simulink library "data_driven_lib_ctl"  (R2024a)
settings: Solver=VariableStepAuto  StartTime=0.0  StopTime=10.0  RelTol=1e-3
undefined symbols (not defined in the file or in its folder): ATDeePC_data, ATDeePC_DT, ATDeePC_LT, ATDeePC_PT, ATDeePC_trajectory_T, ATDeePC_tune_data, ATDeePC_tune_DT, ATDeePC_tune_input_T, ATDeePC_tune_LT, ATDeePC_tune_PT, ATDeePC_tune_trajectory_T, ATExplicitDeePC_data, ATExplicitDeePC_DT, ATExplicitDeePC_PT, DeePC_data, DeePC_DT, DeePC_LT, DeePC_PT, DeePCPI_data, DeePCPI_DT, DeePCPI_LT, DeePCPI_PT, ExplicitDeePC_data, ExplicitDeePC_DT, ExplicitDeePC_PT, ExplicitDeePCCodegen_data, ExplicitDeePCCodegen_DT, ExplicitDeePCCodegen_PT, extrinsic
libraries: otter_controllers x1
settings Model: Creator=luka  LastModifiedBy=luka

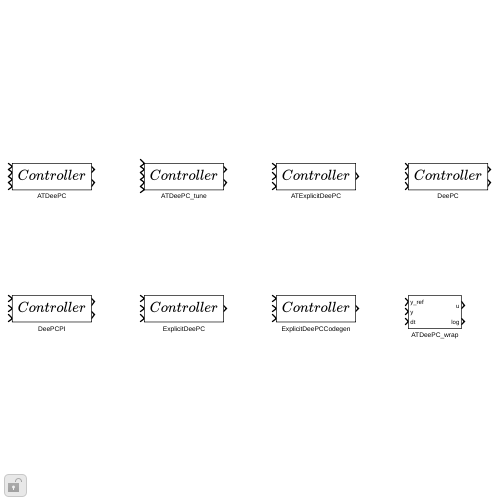
[thumbnail: Simulink's stored preview of the top-level diagram]
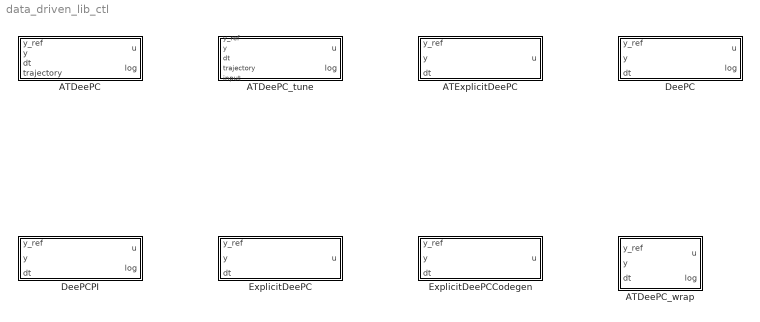
== system data_driven_lib_ctl ==
  ATDeePC : Subsystem  Tag=__cs_comptype:ctl;__cs_compimpl:mat;  mask{iid__=[0], pid__=[65 84 68 101 101 80 67 58 100 97 116 97 95 100 114 105 118 101 110 95 108 105 98], context_path=, params=[], LogEntryType=ATDeePC_LT, data=ATDeePC_data, ParamsType=ATDeePC_PT, DataType=ATDeePC_DT, u_ic=0, trajectory_T=ATDeePC_trajectory_T}
  ATDeePC_tune : Subsystem  Tag=__cs_comptype:ctl;__cs_compimpl:mat;  mask{iid__=[0], pid__=[65 84 68 101 101 80 67 95 116 117 110 101 58 100 97 116 97 95 100 114 105 118 101 110 95 108 105 98], context_path=, params=[], LogEntryType=ATDeePC_tune_LT, data=ATDeePC_tune_data, ParamsType=ATDeePC_tune_PT, DataType=ATDeePC_tune_DT, u_ic=0, trajectory_T=ATDeePC_tune_trajectory_T, input_T=ATDeePC_tune_input_T}
  ATDeePC_wrap : Subsystem  Tag=controller;__cs_comptype:ctl;__cs_compimpl:slx;  mask{trajectory_T=0, data=0, db_params=0, iid__=[0], pid__=[65 84 68 101 101 80 67 95 119 114 97 112 58 100 97 116 97 95 100 114 105 118 101 110 95 108 105 98], context_path=, params=[], params_struct_name=}
  ATExplicitDeePC : Subsystem  Tag=__cs_comptype:ctl;__cs_compimpl:mat;  mask{iid__=[0], pid__=[65 84 69 120 112 108 105 99 105 116 68 101 101 80 67 58 100 97 116 97 95 100 114 105 118 101 110 95 108 105 98], context_path=, params=[], data=ATExplicitDeePC_data, ParamsType=ATExplicitDeePC_PT, DataType=ATExplicitDeePC_DT, u_ic=0}
  DeePC : Subsystem  Tag=__cs_comptype:ctl;__cs_compimpl:mat;  mask{iid__=[0], pid__=[68 101 101 80 67 58 100 97 116 97 95 100 114 105 118 101 110 95 108 105 98], context_path=, params=[], LogEntryType=DeePC_LT, data=DeePC_data, ParamsType=DeePC_PT, DataType=DeePC_DT, u_ic=0}
  DeePCPI : Subsystem  Tag=__cs_comptype:ctl;__cs_compimpl:mat;  mask{iid__=[0], pid__=[68 101 101 80 67 80 73 58 100 97 116 97 95 100 114 105 118 101 110 95 108 105 98], context_path=, params=[], LogEntryType=DeePCPI_LT, data=DeePCPI_data, ParamsType=DeePCPI_PT, DataType=DeePCPI_DT, u_ic=0}
  ExplicitDeePC : Subsystem  Tag=__cs_comptype:ctl;__cs_compimpl:mat;  mask{iid__=[0], pid__=[69 120 112 108 105 99 105 116 68 101 101 80 67 58 100 97 116 97 95 100 114 105 118 101 110 95 108 105 98], context_path=, params=[], data=ExplicitDeePC_data, ParamsType=ExplicitDeePC_PT, DataType=ExplicitDeePC_DT, u_ic=0}
  ExplicitDeePCCodegen : Subsystem  Tag=__cs_comptype:ctl;__cs_compimpl:mat;  mask{iid__=[0], pid__=[69 120 112 108 105 99 105 116 68 101 101 80 67 67 111 100 101 103 101 110 58 100 97 116 97 95 100 114 105 118 101 110 95 108 105 98], context_path=, params=[], data=ExplicitDeePCCodegen_data, ParamsType=ExplicitDeePCCodegen_PT, DataType=ExplicitDeePCCodegen_DT, u_ic=0}

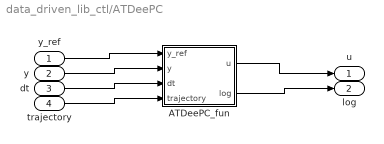
== system data_driven_lib_ctl/ATDeePC ==
  y_ref : Inport
  y : Inport  Port=2
  dt : Inport  Port=3
  trajectory : Inport  Port=4
  ATDeePC_fun : MATLAB Function  TreatAsAtomicUnit=on
  u : Outport
  log : Outport  Port=2
  wires:
  y_ref/1 -> ATDeePC_fun/1(y_ref)
  y/1 -> ATDeePC_fun/2(y)
  dt/1 -> ATDeePC_fun/3(dt)
  trajectory/1 -> ATDeePC_fun/4(trajectory)
  ATDeePC_fun/1(u) -> u/1
  ATDeePC_fun/2(log) -> log/1

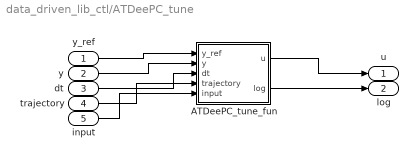
== system data_driven_lib_ctl/ATDeePC_tune ==
  y_ref : Inport
  y : Inport  Port=2
  dt : Inport  Port=3
  trajectory : Inport  Port=4
  input : Inport  Port=5
  ATDeePC_tune_fun : MATLAB Function  TreatAsAtomicUnit=on
  u : Outport
  log : Outport  Port=2
  wires:
  y_ref/1 -> ATDeePC_tune_fun/1(y_ref)
  y/1 -> ATDeePC_tune_fun/2(y)
  dt/1 -> ATDeePC_tune_fun/3(dt)
  trajectory/1 -> ATDeePC_tune_fun/4(trajectory)
  input/1 -> ATDeePC_tune_fun/5(input)
  ATDeePC_tune_fun/1(u) -> u/1
  ATDeePC_tune_fun/2(log) -> log/1

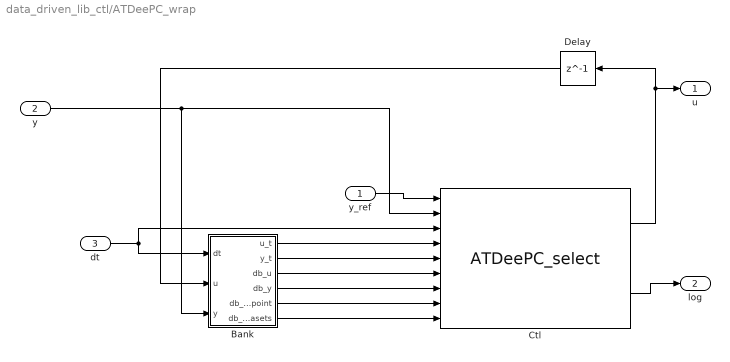
== system data_driven_lib_ctl/ATDeePC_wrap ==
  y_ref : Inport
  y : Inport  Port=2
  dt : Inport  Port=3
  Bank : MATLAB Function  TreatAsAtomicUnit=on
  Ctl : otter_controllers/ATDeePC_select  SystemSampleTime=-1  VariantActivationTime=update diagram  AllowFlexibleInterface=on  Latency=0  AutoFrameSizeCalculation=off
      link override ATDeePC1: params=params.deepc_params
  Delay : Delay  DelayLength=1
  u : Outport
  log : Outport  Port=2
  wires:
  y/1 -> Bank/3(y), Ctl/2
  y_ref/1 -> Ctl/1
  dt/1 -> Bank/1(dt), Ctl/3
  Ctl/1 -> Delay/1, u/1
  Ctl/2 -> log/1
  Delay/1 -> Bank/2(u)
  Bank/1(u_t) -> Ctl/4
  Bank/2(y_t) -> Ctl/5
  Bank/3(db_u) -> Ctl/6
  Bank/4(db_y) -> Ctl/7
  Bank/5(db_endpoint) -> Ctl/8
  Bank/6(db_num_datasets) -> Ctl/9

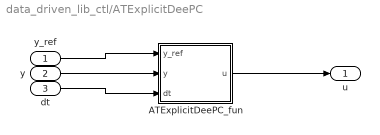
== system data_driven_lib_ctl/ATExplicitDeePC ==
  y_ref : Inport
  y : Inport  Port=2
  dt : Inport  Port=3
  ATExplicitDeePC_fun : MATLAB Function  TreatAsAtomicUnit=on
  u : Outport
  wires:
  y_ref/1 -> ATExplicitDeePC_fun/1(y_ref)
  y/1 -> ATExplicitDeePC_fun/2(y)
  dt/1 -> ATExplicitDeePC_fun/3(dt)
  ATExplicitDeePC_fun/1(u) -> u/1

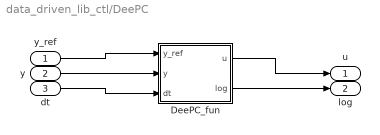
== system data_driven_lib_ctl/DeePC ==
  y_ref : Inport
  y : Inport  Port=2
  dt : Inport  Port=3
  DeePC_fun : MATLAB Function  TreatAsAtomicUnit=on
  u : Outport
  log : Outport  Port=2
  wires:
  y_ref/1 -> DeePC_fun/1(y_ref)
  y/1 -> DeePC_fun/2(y)
  dt/1 -> DeePC_fun/3(dt)
  DeePC_fun/1(u) -> u/1
  DeePC_fun/2(log) -> log/1

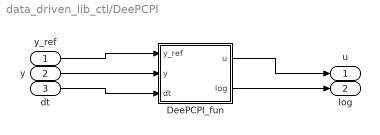
== system data_driven_lib_ctl/DeePCPI ==
  y_ref : Inport
  y : Inport  Port=2
  dt : Inport  Port=3
  DeePCPI_fun : MATLAB Function  TreatAsAtomicUnit=on
  u : Outport
  log : Outport  Port=2
  wires:
  y_ref/1 -> DeePCPI_fun/1(y_ref)
  y/1 -> DeePCPI_fun/2(y)
  dt/1 -> DeePCPI_fun/3(dt)
  DeePCPI_fun/1(u) -> u/1
  DeePCPI_fun/2(log) -> log/1

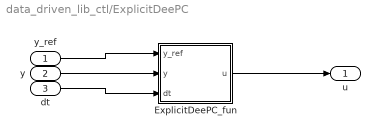
== system data_driven_lib_ctl/ExplicitDeePC ==
  y_ref : Inport
  y : Inport  Port=2
  dt : Inport  Port=3
  ExplicitDeePC_fun : MATLAB Function  TreatAsAtomicUnit=on
  u : Outport
  wires:
  y_ref/1 -> ExplicitDeePC_fun/1(y_ref)
  y/1 -> ExplicitDeePC_fun/2(y)
  dt/1 -> ExplicitDeePC_fun/3(dt)
  ExplicitDeePC_fun/1(u) -> u/1

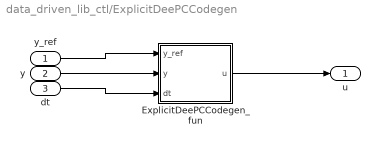
== system data_driven_lib_ctl/ExplicitDeePCCodegen ==
  y_ref : Inport
  y : Inport  Port=2
  dt : Inport  Port=3
  ExplicitDeePCCodegen_fun : MATLAB Function  TreatAsAtomicUnit=on
  u : Outport
  wires:
  y_ref/1 -> ExplicitDeePCCodegen_fun/1(y_ref)
  y/1 -> ExplicitDeePCCodegen_fun/2(y)
  dt/1 -> ExplicitDeePCCodegen_fun/3(dt)
  ExplicitDeePCCodegen_fun/1(u) -> u/1

== matlab function data_driven_lib_ctl/ExplicitDeePC/ExplicitDeePC_fun ==
  settings: updateMethod=DISCRETE
  data: y_ref input; u output; y input; dt input; extrinsic parameter int32; iid__ parameter uint8; pid__ parameter uint8; data parameter DataType; params parameter ParamsType; u_ic parameter double
% __classname:="ExplicitDeePC";
% __lib_name:="data_driven_lib";
% __comp_type:="ctl";
% __plugin_type:="mat";
% __fnname:="fcn_c568dc3885274d46afc145b948c5bd04";
% __input_args:="y_ref, y, dt, u_ic, params, data, pid__, iid__";
% __output_args:=" u";
% __fn_output_args:=" u";
% __ctor_args:="'Params', params, 'Data', data, 'pid', pid__, 'iid', iid__";
% __cfg_args:="u_ic, size(y), size(y_ref)";
% __step_args:="y_ref, y, dt";
function u = fcn(y_ref, y, dt, extrinsic, iid__, pid__, data, params, u_ic)
    coder.extrinsic('fcn_c568dc3885274d46afc145b948c5bd04_ext');
    if extrinsic
u = u_ic;;
         u = fcn_c568dc3885274d46afc145b948c5bd04_ext(y_ref, y, dt, u_ic, params, data, pid__, iid__);
    else
         u = fcn_c568dc3885274d46afc145b948c5bd04(y_ref, y, dt, u_ic, params, data, pid__, iid__);
    end 
end

 
function  u = fcn_c568dc3885274d46afc145b948c5bd04(y_ref, y, dt, u_ic, params, data, pid__, iid__)
    persistent obj
    if isempty(obj)
        obj = ExplicitDeePC('Params', params, 'Data', data, 'pid', pid__, 'iid', iid__);
        obj = obj.configure(u_ic, size(y), size(y_ref));
    end
    [obj,  u] = obj.step(y_ref, y, dt);
    log = eval_log(obj.data);
end

function log = eval_log(data)
        log = 0;

end

== matlab function data_driven_lib_ctl/ExplicitDeePCCodegen/ExplicitDeePCCodegen_fun ==
  settings: updateMethod=DISCRETE
  data: y_ref input; u output; y input; dt input; extrinsic parameter int32; iid__ parameter uint8; pid__ parameter uint8; data parameter DataType; params parameter ParamsType; u_ic parameter double
% __classname:="ExplicitDeePCCodegen";
% __lib_name:="data_driven_lib";
% __comp_type:="ctl";
% __plugin_type:="mat";
% __fnname:="fcn_376b43e32e9244da81b041186f99c4c2";
% __input_args:="y_ref, y, dt, u_ic, params, data, pid__, iid__";
% __output_args:=" u";
% __fn_output_args:=" u";
% __ctor_args:="'Params', params, 'Data', data, 'pid', pid__, 'iid', iid__";
% __cfg_args:="u_ic, size(y), size(y_ref)";
% __step_args:="y_ref, y, dt";
function u = fcn(y_ref, y, dt, extrinsic, iid__, pid__, data, params, u_ic)
    coder.extrinsic('fcn_376b43e32e9244da81b041186f99c4c2_ext');
    if extrinsic
u = u_ic;;
         u = fcn_376b43e32e9244da81b041186f99c4c2_ext(y_ref, y, dt, u_ic, params, data, pid__, iid__);
    else
         u = fcn_376b43e32e9244da81b041186f99c4c2(y_ref, y, dt, u_ic, params, data, pid__, iid__);
    end 
end

 
function  u = fcn_376b43e32e9244da81b041186f99c4c2(y_ref, y, dt, u_ic, params, data, pid__, iid__)
    persistent obj
    if isempty(obj)
        obj = ExplicitDeePCCodegen('Params', params, 'Data', data, 'pid', pid__, 'iid', iid__);
        obj = obj.configure(u_ic, size(y), size(y_ref));
    end
    [obj,  u] = obj.step(y_ref, y, dt);
    log = eval_log(obj.data);
end

function log = eval_log(data)
        log = 0;

end

== matlab function data_driven_lib_ctl/ATDeePC_wrap/Bank ==
  settings: updateMethod=DISCRETE
  data: u_t output; y_t output; dt input; db_u output; u input; y input; db_params parameter; data parameter; db_y output; db_endpoint output; db_num_datasets output
function [u_t, y_t, db_u, db_y, db_endpoint, db_num_datasets] = fcn(dt, u, y, db_params, data)

    persistent t u_traj y_traj last_changed_t db_u_p db_y_p db_endpoint_p db_num_datasets_p    

    traj_len = data.T;
    if isempty(t)
        t = 0;
        last_changed_t = 0;
        db_num_datasets_p = db_params.num_datasets_in_bank;
        db_u_p = zeros(db_params.dataset_bank_size, data.T, data.m);
        db_y_p = zeros(db_params.dataset_bank_size, data.T, data.p);
        db_endpoint_p = zeros(db_params.dataset_bank_size, data.m);
        if db_num_datasets_p > 0
            db_u_p(end-db_num_datasets_p+1, :, :) = db_params.D_u;
            db_y_p(end-db_num_datasets_p+1, :, :) = db_params.D_y;
            db_endpoint_p(end-db_num_datasets_p+1, :, :) = db_params.end_point;
        end
        u_traj = zeros(traj_len, data.m);
        y_traj = zeros(traj_len, data.p);
    end

    t = t + dt;

    coder.extrinsic('trajectory_dataset'); % arx function not supported
    u_traj = circshift(u_traj, -1);
    y_traj = circshift(y_traj, -1);
    u_traj(end, :) = u(db_params.input_record_dims);
    y_traj(end, :) = y(db_params.output_record_dims);

    u_t = u_traj;
    y_t = y_traj;    
    
    
    [t, last_changed_t, db_u_p, db_y_p, db_endpoint_p, db_num_datasets_p, ...
       db_u, db_y, db_endpoint, db_num_datasets] = ...
          update_dataset_bank(t, last_changed_t, db_u_p, db_y_p, db_endpoint_p, db_num_datasets_p, dt, u_traj, y_traj, db_params, data);

end

== matlab function data_driven_lib_ctl/ATDeePC_tune/ATDeePC_tune_fun ==
  settings: updateMethod=DISCRETE
  data: y_ref input; u output; y input; dt input; trajectory input trajectory_T; input input input_T; log output LogEntryType; extrinsic parameter int32; iid__ parameter uint8; pid__ parameter uint8; data parameter DataType; params parameter ParamsType; u_ic parameter double
% __classname:="ATDeePC_tune";
% __lib_name:="data_driven_lib";
% __comp_type:="ctl";
% __plugin_type:="mat";
% __fnname:="fcn_5beb4988f2a54aae89cc0e73a28b2e2c";
% __input_args:="y_ref, y, dt, trajectory, input, u_ic, params, data, pid__, iid__";
% __output_args:=" u";
% __fn_output_args:="u, log";
% __ctor_args:="'Params', params, 'Data', data, 'pid', pid__, 'iid', iid__";
% __cfg_args:="u_ic, size(y), size(y_ref)";
% __step_args:="y_ref, y, dt, trajectory, input";
function [  u, log] = fcn(y_ref, y, dt, trajectory, input, extrinsic, iid__, pid__, data, params, u_ic)
    coder.extrinsic('fcn_5beb4988f2a54aae89cc0e73a28b2e2c_ext');
    if extrinsic
u = u_ic;;
        [  u, log] = fcn_5beb4988f2a54aae89cc0e73a28b2e2c_ext(y_ref, y, dt, trajectory, input, u_ic, params, data, pid__, iid__);
    else
        [  u, log] = fcn_5beb4988f2a54aae89cc0e73a28b2e2c(y_ref, y, dt, trajectory, input, u_ic, params, data, pid__, iid__);
    end 
end

 
function [  u, log] = fcn_5beb4988f2a54aae89cc0e73a28b2e2c(y_ref, y, dt, trajectory, input, u_ic, params, data, pid__, iid__)
    persistent obj
    if isempty(obj)
        obj = ATDeePC_tune('Params', params, 'Data', data, 'pid', pid__, 'iid', iid__);
        obj = obj.configure(u_ic, size(y), size(y_ref));
    end
    [obj,  u] = obj.step(y_ref, y, dt, trajectory, input);
    log = eval_log(obj.data);
end

function log = eval_log(data)
        log.x_op_u = double(data.x_op_u);
    log.x_op_y = double(data.x_op_y);
    log.x_op_g = double(data.x_op_g);

end

== matlab function data_driven_lib_ctl/ATDeePC/ATDeePC_fun ==
  settings: updateMethod=DISCRETE
  data: y_ref input; u output; y input; dt input; trajectory input trajectory_T; log output LogEntryType; extrinsic parameter int32; iid__ parameter uint8; pid__ parameter uint8; data parameter DataType; params parameter ParamsType; u_ic parameter double
% __classname:="ATDeePC";
% __lib_name:="data_driven_lib";
% __comp_type:="ctl";
% __plugin_type:="mat";
% __fnname:="fcn_2264c8080b8942408004d7261a82db6c";
% __input_args:="y_ref, y, dt, trajectory, u_ic, params, data, pid__, iid__";
% __output_args:=" u";
% __fn_output_args:="u, log";
% __ctor_args:="'Params', params, 'Data', data, 'pid', pid__, 'iid', iid__";
% __cfg_args:="u_ic, size(y), size(y_ref)";
% __step_args:="y_ref, y, dt, trajectory";
function [  u, log] = fcn(y_ref, y, dt, trajectory, extrinsic, iid__, pid__, data, params, u_ic)
    coder.extrinsic('fcn_2264c8080b8942408004d7261a82db6c_ext');
    if extrinsic
u = u_ic;;
        [  u, log] = fcn_2264c8080b8942408004d7261a82db6c_ext(y_ref, y, dt, trajectory, u_ic, params, data, pid__, iid__);
    else
        [  u, log] = fcn_2264c8080b8942408004d7261a82db6c(y_ref, y, dt, trajectory, u_ic, params, data, pid__, iid__);
    end 
end

 
function [  u, log] = fcn_2264c8080b8942408004d7261a82db6c(y_ref, y, dt, trajectory, u_ic, params, data, pid__, iid__)
    persistent obj
    if isempty(obj)
        obj = ATDeePC('Params', params, 'Data', data, 'pid', pid__, 'iid', iid__);
        obj = obj.configure(u_ic, size(y), size(y_ref));
    end
    [obj,  u] = obj.step(y_ref, y, dt, trajectory);
    log = eval_log(obj.data);
end

function log = eval_log(data)
        log.x_op_u = double(data.x_op_u);
    log.x_op_y = double(data.x_op_y);
    log.x_op_g = double(data.x_op_g);

end

== matlab function data_driven_lib_ctl/ATExplicitDeePC/ATExplicitDeePC_fun ==
  settings: updateMethod=DISCRETE
  data: y_ref input; u output; y input; dt input; extrinsic parameter int32; iid__ parameter uint8; pid__ parameter uint8; data parameter DataType; params parameter ParamsType; u_ic parameter double
% __classname:="ATExplicitDeePC";
% __lib_name:="data_driven_lib";
% __comp_type:="ctl";
% __plugin_type:="mat";
% __fnname:="fcn_3d720a34a98b4a66bf956a8e8c46a416";
% __input_args:="y_ref, y, dt, u_ic, params, data, pid__, iid__";
% __output_args:=" u";
% __fn_output_args:=" u";
% __ctor_args:="'Params', params, 'Data', data, 'pid', pid__, 'iid', iid__";
% __cfg_args:="u_ic, size(y), size(y_ref)";
% __step_args:="y_ref, y, dt";
function u = fcn(y_ref, y, dt, extrinsic, iid__, pid__, data, params, u_ic)
    coder.extrinsic('fcn_3d720a34a98b4a66bf956a8e8c46a416_ext');
    if extrinsic
u = u_ic;;
         u = fcn_3d720a34a98b4a66bf956a8e8c46a416_ext(y_ref, y, dt, u_ic, params, data, pid__, iid__);
    else
         u = fcn_3d720a34a98b4a66bf956a8e8c46a416(y_ref, y, dt, u_ic, params, data, pid__, iid__);
    end 
end

 
function  u = fcn_3d720a34a98b4a66bf956a8e8c46a416(y_ref, y, dt, u_ic, params, data, pid__, iid__)
    persistent obj
    if isempty(obj)
        obj = ATExplicitDeePC('Params', params, 'Data', data, 'pid', pid__, 'iid', iid__);
        obj = obj.configure(u_ic, size(y), size(y_ref));
    end
    [obj,  u] = obj.step(y_ref, y, dt);
    log = eval_log(obj.data);
end

function log = eval_log(data)
        log = 0;

end

== matlab function data_driven_lib_ctl/DeePC/DeePC_fun ==
  settings: updateMethod=DISCRETE
  data: y_ref input; u output; y input; dt input; log output LogEntryType; extrinsic parameter int32; iid__ parameter uint8; pid__ parameter uint8; data parameter DataType; params parameter ParamsType; u_ic parameter double
% __classname:="DeePC";
% __lib_name:="data_driven_lib";
% __comp_type:="ctl";
% __plugin_type:="mat";
% __fnname:="fcn_0842399a477542d4b8b1d5ac5da99eb0";
% __input_args:="y_ref, y, dt, u_ic, params, data, pid__, iid__";
% __output_args:=" u";
% __fn_output_args:="u, log";
% __ctor_args:="'Params', params, 'Data', data, 'pid', pid__, 'iid', iid__";
% __cfg_args:="u_ic, size(y), size(y_ref)";
% __step_args:="y_ref, y, dt";
function [  u, log] = fcn(y_ref, y, dt, extrinsic, iid__, pid__, data, params, u_ic)
    coder.extrinsic('fcn_0842399a477542d4b8b1d5ac5da99eb0_ext');
    if extrinsic
u = u_ic;;
        [  u, log] = fcn_0842399a477542d4b8b1d5ac5da99eb0_ext(y_ref, y, dt, u_ic, params, data, pid__, iid__);
    else
        [  u, log] = fcn_0842399a477542d4b8b1d5ac5da99eb0(y_ref, y, dt, u_ic, params, data, pid__, iid__);
    end 
end

 
function [  u, log] = fcn_0842399a477542d4b8b1d5ac5da99eb0(y_ref, y, dt, u_ic, params, data, pid__, iid__)
    persistent obj
    if isempty(obj)
        obj = DeePC('Params', params, 'Data', data, 'pid', pid__, 'iid', iid__);
        obj = obj.configure(u_ic, size(y), size(y_ref));
    end
    [obj,  u] = obj.step(y_ref, y, dt);
    log = eval_log(obj.data);
end

function log = eval_log(data)
        log.x_op_u = double(data.x_op_u);
    log.x_op_y = double(data.x_op_y);
    log.x_op_g = double(data.x_op_g);

end

== matlab function data_driven_lib_ctl/DeePCPI/DeePCPI_fun ==
  settings: updateMethod=DISCRETE
  data: y_ref input; u output; y input; dt input; log output LogEntryType; extrinsic parameter int32; iid__ parameter uint8; pid__ parameter uint8; data parameter DataType; params parameter ParamsType; u_ic parameter double
% __classname:="DeePCPI";
% __lib_name:="data_driven_lib";
% __comp_type:="ctl";
% __plugin_type:="mat";
% __fnname:="fcn_cf9850b8b6f44390a4ebfac3fa4f0666";
% __input_args:="y_ref, y, dt, u_ic, params, data, pid__, iid__";
% __output_args:=" u";
% __fn_output_args:="u, log";
% __ctor_args:="'Params', params, 'Data', data, 'pid', pid__, 'iid', iid__";
% __cfg_args:="u_ic, size(y), size(y_ref)";
% __step_args:="y_ref, y, dt";
function [  u, log] = fcn(y_ref, y, dt, extrinsic, iid__, pid__, data, params, u_ic)
    coder.extrinsic('fcn_cf9850b8b6f44390a4ebfac3fa4f0666_ext');
    if extrinsic
u = u_ic;;
        [  u, log] = fcn_cf9850b8b6f44390a4ebfac3fa4f0666_ext(y_ref, y, dt, u_ic, params, data, pid__, iid__);
    else
        [  u, log] = fcn_cf9850b8b6f44390a4ebfac3fa4f0666(y_ref, y, dt, u_ic, params, data, pid__, iid__);
    end 
end

 
function [  u, log] = fcn_cf9850b8b6f44390a4ebfac3fa4f0666(y_ref, y, dt, u_ic, params, data, pid__, iid__)
    persistent obj
    if isempty(obj)
        obj = DeePCPI('Params', params, 'Data', data, 'pid', pid__, 'iid', iid__);
        obj = obj.configure(u_ic, size(y), size(y_ref));
    end
    [obj,  u] = obj.step(y_ref, y, dt);
    log = eval_log(obj.data);
end

function log = eval_log(data)
        log.x_op_u = double(data.x_op_u);
    log.x_op_y = double(data.x_op_y);
    log.x_op_g = double(data.x_op_g);

end
